simulink model "Stanza_Smart_Lib5"  (R2025a)
settings: Solver=ode4  StartTime=0.0  StopTime=86400  FixedStep=0.01  RelTol=1e-3
values from neighbouring files (symbols this model uses):
  C_aria_Corr = 100000    [setup_casa_smart.m]
  C_muri_Corr = 25000000    [setup_casa_smart.m]
  Coeff_Finestra = 100    [setup_casa_smart.m]
  Deadband = 0.5    [setup_casa_smart.m]
  dt = 0.1    [setup_casa_smart.m]
  Kd = 6000    [setup_casa_smart.m]
  Ki = 0.005    [setup_casa_smart.m]
  Kp = 100    [setup_casa_smart.m]
  P_max = 1200    [setup_casa_smart.m]
  R_ext_Corr = 0.15    [setup_casa_smart.m]
  R_ia = 0.1    [setup_casa_smart.m]
  R_int = 2.0    (= 2)    [setup_casa_smart.m]
  Soglia_Accensione_AC = 24.5    [setup_casa_smart.m]
  Soglia_Apertura_Finestra = 23.5    [setup_casa_smart.m]
  T_start_real = temp_values(1)    [fetch_meteo.m]    (also in setup_casa_smart.m = 20)
libraries: simulink x4
settings Model: Creator=smant  LastModifiedBy=smant
settings OptimizationCC: ZeroExternalMemoryAtStartup=off  ZeroInternalMemoryAtStartup=off
settings RTWCC: GenCodeOnly=on  TargetLang=C++
settings GRTTargetCC: TargetLangStandard=C++11 (ISO)  MatFileLogging=off  CodeInterfacePackaging=C++ class  SubcomponentCodeInterfacePackaging=C++ class

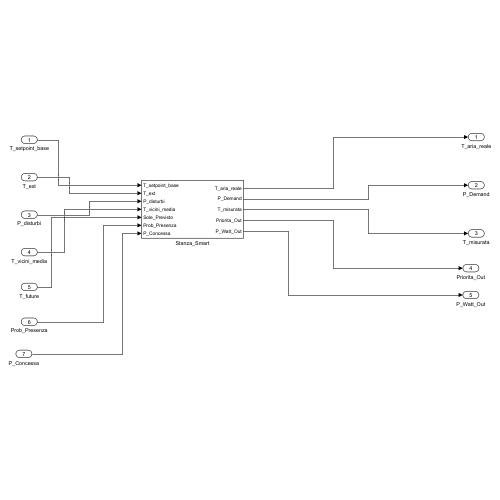
[thumbnail: Simulink's stored preview of the top-level diagram]
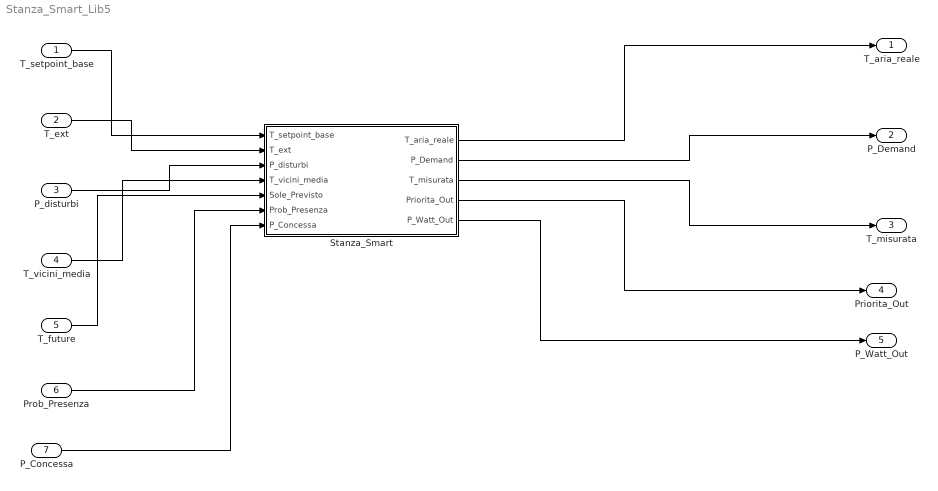
== system Stanza_Smart_Lib5 ==
  T_setpoint_base : Inport
  T_ext : Inport  Port=2
  P_disturbi : Inport  Port=3
  T_vicini_media : Inport  Port=4
  T_future : Inport  Port=5
  Prob_Presenza : Inport  Port=6
  P_Concessa : Inport  Port=7
  Stanza_Smart : Subsystem
  T_aria_reale : Outport
  P_Demand : Outport  Port=2
  T_misurata : Outport  Port=3
  Priorita_Out : Outport  Port=4
  P_Watt_Out : Outport  Port=5
  wires:
  T_setpoint_base/1 -> Stanza_Smart/1(T_setpoint_base)
  P_disturbi/1 -> Stanza_Smart/3(P_disturbi)
  T_ext/1 -> Stanza_Smart/2(T_ext)
  T_vicini_media/1 -> Stanza_Smart/4(T_vicini_media)
  Stanza_Smart/1(T_aria_reale) -> T_aria_reale/1
  Stanza_Smart/3(T_misurata) -> T_misurata/1
  Stanza_Smart/2(P_Demand) -> P_Demand/1
  T_future/1 -> Stanza_Smart/5(Sole_Previsto)
  Stanza_Smart/4(Priorita_Out) -> Priorita_Out/1
  Prob_Presenza/1 -> Stanza_Smart/6(Prob_Presenza)
  P_Concessa/1 -> Stanza_Smart/7(P_Concessa)
  Stanza_Smart/5(P_Watt_Out) -> P_Watt_Out/1

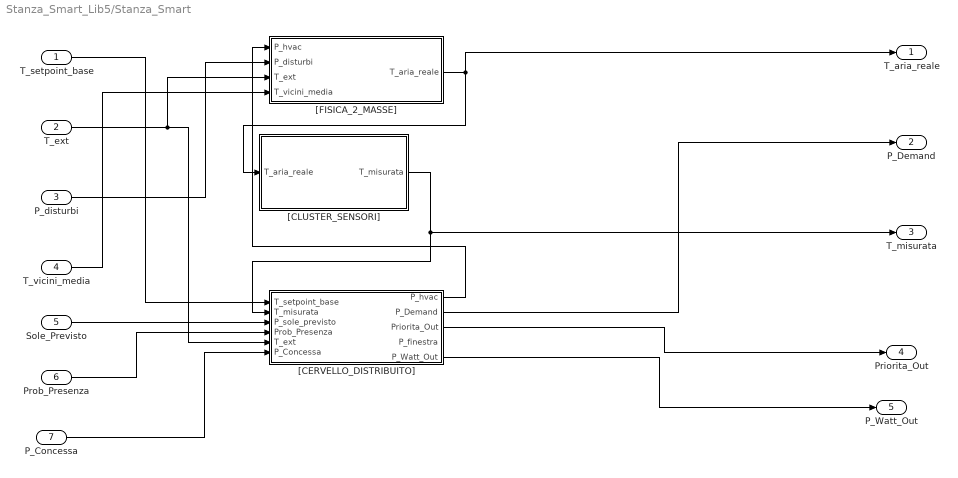
== system Stanza_Smart_Lib5/Stanza_Smart ==
  T_setpoint_base : Inport
  T_ext : Inport  Port=2
  P_disturbi : Inport  Port=3
  T_vicini_media : Inport  Port=4
  Sole_Previsto : Inport  Port=5
  Prob_Presenza : Inport  Port=6
  P_Concessa : Inport  Port=7
  "[CERVELLO_DISTRIBUITO]" : Subsystem
  "[CLUSTER_SENSORI]" : Subsystem
  "[FISICA_2_MASSE]" : Subsystem
  T_aria_reale : Outport
  P_Demand : Outport  Port=2
  T_misurata : Outport  Port=3
  Priorita_Out : Outport  Port=4
  P_Watt_Out : Outport  Port=5
  wires:
  "[CERVELLO_DISTRIBUITO]"/2(P_Demand) -> P_Demand/1
  "[FISICA_2_MASSE]"/1(T_aria_reale) -> T_aria_reale/1, "[CLUSTER_SENSORI]"/1(T_aria_reale)
  "[CLUSTER_SENSORI]"/1(T_misurata) -> T_misurata/1, "[CERVELLO_DISTRIBUITO]"/2(T_misurata)
  T_vicini_media/1 -> "[FISICA_2_MASSE]"/4(T_vicini_media)
  T_setpoint_base/1 -> "[CERVELLO_DISTRIBUITO]"/1(T_setpoint_base)
  T_ext/1 -> "[CERVELLO_DISTRIBUITO]"/5(T_ext), "[FISICA_2_MASSE]"/3(T_ext)
  "[CERVELLO_DISTRIBUITO]"/1(P_hvac) -> "[FISICA_2_MASSE]"/1(P_hvac)
  P_disturbi/1 -> "[FISICA_2_MASSE]"/2(P_disturbi)
  Sole_Previsto/1 -> "[CERVELLO_DISTRIBUITO]"/3(P_sole_previsto)
  "[CERVELLO_DISTRIBUITO]"/3(Priorita_Out) -> Priorita_Out/1
  Prob_Presenza/1 -> "[CERVELLO_DISTRIBUITO]"/4(Prob_Presenza)
  P_Concessa/1 -> "[CERVELLO_DISTRIBUITO]"/6(P_Concessa)
  "[CERVELLO_DISTRIBUITO]"/5(P_Watt_Out) -> P_Watt_Out/1

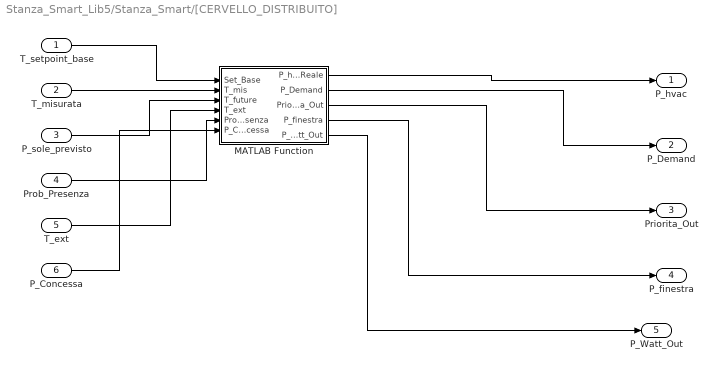
== system Stanza_Smart_Lib5/Stanza_Smart/[CERVELLO_DISTRIBUITO] ==
  T_setpoint_base : Inport
  T_misurata : Inport  Port=2
  P_sole_previsto : Inport  Port=3
  Prob_Presenza : Inport  Port=4
  T_ext : Inport  Port=5
  P_Concessa : Inport  Port=6
  MATLAB Function : MATLAB Function  TreatAsAtomicUnit=on
  P_hvac : Outport
  P_Demand : Outport  Port=2
  Priorita_Out : Outport  Port=3
  P_finestra : Outport  Port=4
  P_Watt_Out : Outport  Port=5
  wires:
  MATLAB Function/1(P_hvac_Reale) -> P_hvac/1
  T_setpoint_base/1 -> MATLAB Function/1(Set_Base)
  T_misurata/1 -> MATLAB Function/2(T_mis)
  P_sole_previsto/1 -> MATLAB Function/3(T_future)
  Prob_Presenza/1 -> MATLAB Function/5(Prob_Presenza)
  T_ext/1 -> MATLAB Function/4(T_ext)
  MATLAB Function/4(P_finestra) -> P_finestra/1
  MATLAB Function/3(Priorita_Out) -> Priorita_Out/1
  MATLAB Function/2(P_Demand) -> P_Demand/1
  P_Concessa/1 -> MATLAB Function/6(P_Concessa)
  MATLAB Function/5(P_Watt_Out) -> P_Watt_Out/1

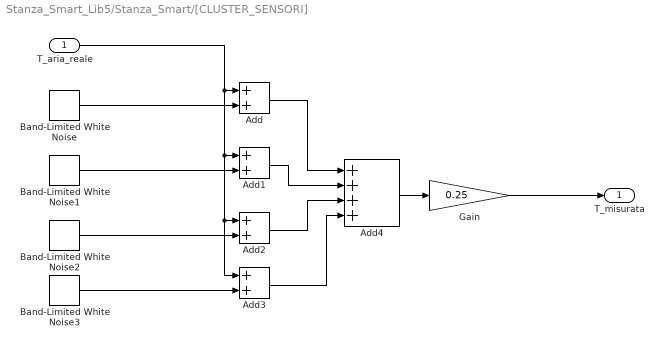
== system Stanza_Smart_Lib5/Stanza_Smart/[CLUSTER_SENSORI] ==
  T_aria_reale : Inport
  Add{,1..3} (4 alike) : Sum
  Add4 : Sum  Inputs=++++
  Band-Limited White Noise : simulink/Sources/Band-Limited White Noise  Cov=0  Ts=0.1  seed=1
  Band-Limited White Noise1 : simulink/Sources/Band-Limited White Noise  Cov=0  Ts=0.1  seed=2
  Band-Limited White Noise2 : simulink/Sources/Band-Limited White Noise  Cov=0  Ts=0.1  seed=3
  Band-Limited White Noise3 : simulink/Sources/Band-Limited White Noise  Cov=0  Ts=0.1  seed=4
  Gain : Gain  Gain=0.25
  T_misurata : Outport
  wires:
  T_aria_reale/1 -> Add3/1, Add2/1, Add1/1, Add/1
  Band-Limited White Noise/1 -> Add/2
  Band-Limited White Noise1/1 -> Add1/2
  Band-Limited White Noise2/1 -> Add2/2
  Band-Limited White Noise3/1 -> Add3/2
  Add/1 -> Add4/1
  Add1/1 -> Add4/2
  Add2/1 -> Add4/3
  Add3/1 -> Add4/4
  Add4/1 -> Gain/1
  Gain/1 -> T_misurata/1

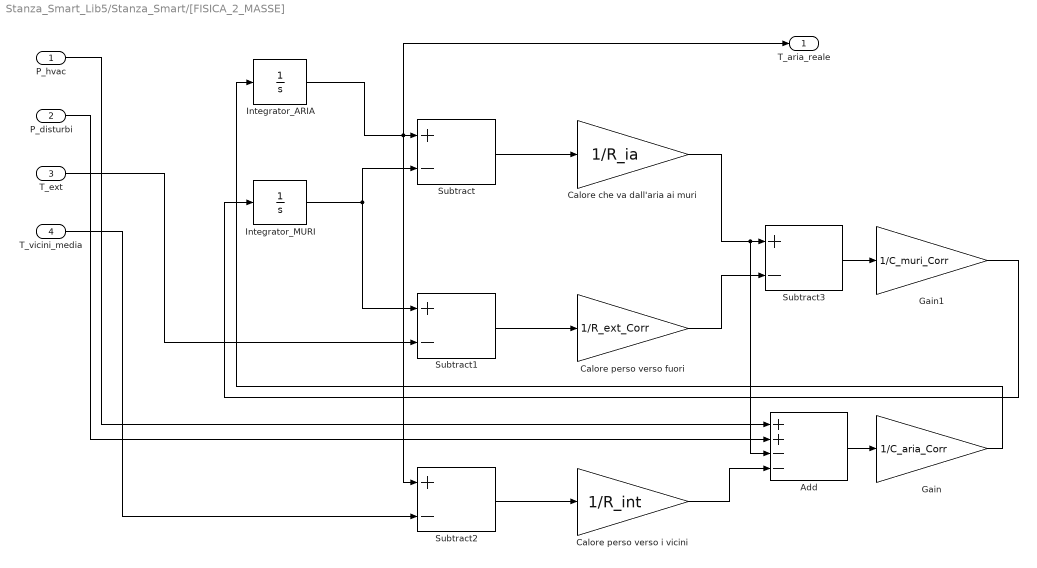
== system Stanza_Smart_Lib5/Stanza_Smart/[FISICA_2_MASSE] ==
  P_hvac : Inport
  P_disturbi : Inport  Port=2
  T_ext : Inport  Port=3
  T_vicini_media : Inport  Port=4
  Add : Sum  Inputs=++--
  Calore che va dall'aria ai muri : Gain  Gain=1/R_ia
  Calore perso verso fuori : Gain  Gain=1/R_ext_Corr
  Calore perso verso i vicini : Gain  Gain=1/R_int
  Gain : Gain  Gain=1/C_aria_Corr
  Gain1 : Gain  Gain=1/C_muri_Corr
  Integrator_ARIA : Integrator  InitialCondition=T_start_real
  Integrator_MURI : Integrator  InitialCondition=T_start_real
  Subtract{,1..3} (4 alike) : Sum  Inputs=+-
  T_aria_reale : Outport
  wires:
  Integrator_ARIA/1 -> Subtract2/1, Subtract/1, T_aria_reale/1
  Integrator_MURI/1 -> Subtract1/1, Subtract/2
  T_ext/1 -> Subtract1/2
  Subtract/1 -> Calore che va dall'aria ai muri/1
  Subtract1/1 -> Calore perso verso fuori/1
  T_vicini_media/1 -> Subtract2/2
  Subtract2/1 -> Calore perso verso i vicini/1
  Calore che va dall'aria ai muri/1 -> Add/3, Subtract3/1
  Calore perso verso fuori/1 -> Subtract3/2
  Subtract3/1 -> Gain1/1
  Gain1/1 -> Integrator_MURI/1
  P_hvac/1 -> Add/1
  P_disturbi/1 -> Add/2
  Calore perso verso i vicini/1 -> Add/4
  Add/1 -> Gain/1
  Gain/1 -> Integrator_ARIA/1

== matlab function Stanza_Smart_Lib5/Stanza_Smart/[CERVELLO_DISTRIBUITO]/MATLAB Function ==
  settings: updateMethod=DISCRETE  sampleTime=0.1
  data: Set_Base input; T_mis input; T_future input; T_ext input; Kp parameter; Ki parameter; P_max parameter; P_hvac_Reale output; dt parameter; Deadband parameter; Kd parameter; Coeff_Finestra parameter; Soglia_Apertura_Finestra parameter; Soglia_Accensione_AC parameter; Prob_Presenza input; P_Demand output; Priorita_Out output; P_finestra output; P_Concessa input; P_Watt_Out output
function [P_hvac_Reale, P_Demand, Priorita_Out, P_finestra, P_Watt_Out] = fcn(Set_Base, T_mis, T_future, T_ext, Kp, Ki, P_max, dt, Deadband, Kd, Coeff_Finestra, Soglia_Apertura_Finestra, Soglia_Accensione_AC, Prob_Presenza, P_Concessa)
%#codegen
% CERVELLO DISTRIBUITO V3: 
% PID + Isteresi + Finestra + Consenso + Rampa + OUTPUT CONSUMO DIRETTO

% --- MEMORIA ---
persistent Integral_Error Prev_Error Window_State Heating_State Prev_P_hvac;

if isempty(Integral_Error)
    Integral_Error = 0;
    Prev_Error = 0;
    Window_State = 0; 
    Heating_State = 1; 
    Prev_P_hvac = 0; 
end

% =========================================================
% 1. TARGETING (Setpoint)
% =========================================================
Target = Set_Base;

% Logica Meteo (Protezione Gelo)
if (Set_Base < 20) && (T_future < 2.0)
    Target = max(Target, 19.0);
end

% =========================================================
% 2. GESTIONE FINESTRA
% =========================================================
Isteresi_Finestra = 0.5; 
if (T_mis > Soglia_Apertura_Finestra) && (T_ext < T_mis)
    Window_State = 1;
elseif T_mis < (Soglia_Apertura_Finestra - Isteresi_Finestra)
    Window_State = 0;
end

if Window_State == 1
    P_finestra = Coeff_Finestra * (T_ext - T_mis);
else
    P_finestra = 0;
end

% =========================================================
% 3. LOGICA ISTERESI (ON/OFF)
% =========================================================
Soglia_Spegni = Target + Deadband; 
Soglia_Accendi = Target;           

if Heating_State == 1
    if T_mis >= Soglia_Spegni
        Heating_State = 0; 
    end
else
    if T_mis <= Soglia_Accendi
        Heating_State = 1; 
    end
end

% =========================================================
% 4. CALCOLO PID (La Domanda Ideale)
% =========================================================
Errore = Target - T_mis;

if Heating_State == 0
    P_calc = 0;
    Integral_Error = 0; 
    Prev_Error = 0;
else
    P_term = Errore * Kp;
    
    Integral_Error = Integral_Error + (Errore * dt);
    Limit_Int = P_max / Ki; 
    if Integral_Error > Limit_Int, Integral_Error = Limit_Int;
    elseif Integral_Error < -Limit_Int, Integral_Error = -Limit_Int;
    end
    I_term = Integral_Error * Ki;
    
    Derivative = (Errore - Prev_Error) / dt;
    D_term = Derivative * Kd;
    
    P_calc = P_term + I_term + D_term;
    Prev_Error = Errore;
end

% =========================================================
% 5. GESTIONE DOMANDA vs CONCESSIONE
% =========================================================
Min_Power = 200; 
P_Ideal = 0;

% A. Calcolo della Domanda Ideale
if P_calc > 0
    % Riscaldamento
    if P_calc < Min_Power
        P_Ideal = 0; 
    elseif P_calc > P_max
        P_Ideal = P_max;
    else
        P_Ideal = P_calc;
    end
else
    % Raffreddamento (AC)
    if T_mis > Soglia_Accensione_AC
        if abs(P_calc) < Min_Power
             P_Ideal = 0;
        elseif P_calc < -P_max
            P_Ideal = -P_max;
        else
            P_Ideal = P_calc;
        end
    else
        P_Ideal = 0;
    end
end

% OUTPUT VERSO IL GESTORE CENTRALE
P_Demand = P_Ideal;
Priorita_Out = Prob_Presenza;

% B. Applicazione del Limite Concesso
Limit_Abs = abs(P_Concessa);

if P_Ideal > 0
    P_Final_Target = min(P_Ideal, Limit_Abs);
else
    if abs(P_Ideal) > Limit_Abs
        P_Final_Target = -Limit_Abs;
    else
        P_Final_Target = P_Ideal;
    end
end

% =========================================================
% 6. RAMPA SOFT-START & OUTPUT CONSUMI
% =========================================================
Max_Change_Per_Second = 2.0; 
Max_Step = Max_Change_Per_Second * dt; 

Delta = P_Final_Target - Prev_P_hvac;

if abs(Delta) > Max_Step
    if Delta > 0
        P_hvac_Reale = Prev_P_hvac + Max_Step;
    else
        P_hvac_Reale = Prev_P_hvac - Max_Step;
    end
else
    P_hvac_Reale = P_Final_Target;
end

Prev_P_hvac = P_hvac_Reale;

% --- CONVERSIONE CONSUMI INTERNA ---
% Restituisce il valore assoluto (sempre positivo) per il contatore
P_Watt_Out = abs(P_hvac_Reale);
